simulink model "pressingswitch_fan_stateflow_experiment"  (R2021a)
settings: Solver=VariableStepAuto  StartTime=0.0  StopTime=11  RelTol=1e-3
settings Model: Creator=surya  LastModifiedBy=surya

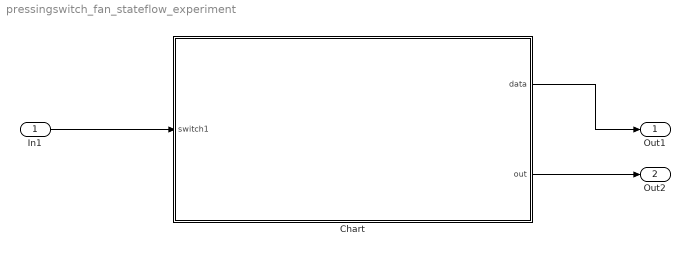
== system pressingswitch_fan_stateflow_experiment ==
  In1 : Inport
  Chart : Stateflow chart  TreatAsAtomicUnit=on
  Out1 : Outport
  Out2 : Outport  Port=2
  wires:
  Chart/1(data) -> Out1/1
  Chart/2(out) -> Out2/1
  In1/1 -> Chart/1(switch1)

== stateflow chart pressingswitch_fan_stateflow_experiment/Chart ==
  state counter2(y) [function]
    (default) -> (junction 2)
    (junction 2) -> (junction 1) : {t=y}
    (junction 1) -> (junction 3) [order 1] : [switch1==1& t<500]
    (junction 4) -> (junction 1)
    (junction 1) -> (junction 5) [order 2] : {data=t}
    (junction 3) -> (junction 4) : {t=t+1}
  state off
    en:
    out=0
  state on
    en:
    out=1
  (default) -> off
  off -> (junction 28) : [switch1==1]{counter2(0)}
  (junction 28) -> on : [switch1==1& data>=500]
  on -> off : [switch1==0]
  data: y function_input; data output; t local; out output; switch1 input
